simulink model "task4_lab10"  (R2021a)
settings: Solver=FixedStepDiscrete  StartTime=0.0  StopTime=10.0  RelTol=1e-3
settings Model: Creator=reemb  LastModifiedBy=reemb
settings OptimizationCC: DefaultParameterBehavior=Inlined  EnhancedBackFolding=on  PassReuseOutputArgsAs=Individual arguments  ZeroExternalMemoryAtStartup=off  ZeroInternalMemoryAtStartup=off  OptimizeBlockOrder=speed  DifferentSizesBufferReuse=on  OptimizationCustomize=off  EfficientTunableParamExpr=on
settings DebuggingCC: ParameterTunabilityLossMsg=error
settings SFSimCC: MATLABDynamicMemAlloc=off
settings RTWCC: SystemTargetFile=ert.tlc  GenCodeOnly=on  TemplateMakefile=ert_default_tmf
settings CodeAppCC: ForceParamTrailComments=on  IgnoreCustomStorageClasses=off  OperatorAnnotations=on  SimulinkDataObjDesc=on  SFDataObjDesc=on  InsertBlockDesc=on
settings ERTTargetCC: TargetLangStandard=C99 (ISO)  GenerateSampleERTMain=on  InlinedParameterPlacement=NonHierarchical  ERTCustomFileTemplate=example_file_process.tlc

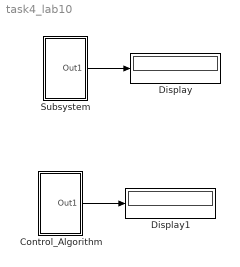
== system task4_lab10 ==
  Control_Algorithm : Subsystem  TreatAsAtomicUnit=on  RTWFcnName=algo_logic
      settings: RTWSystemCode=Nonreusable function  RTWFcnNameOpts=User specified  RTWFileNameOpts=Use function name
  Display : Display
  Display1 : Display
  Subsystem : Subsystem
  wires:
  Subsystem/1(Out1) -> Display/1
  Control_Algorithm/1(Out1) -> Display1/1

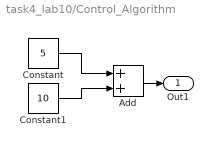
== system task4_lab10/Control_Algorithm ==
  Add : Sum
  Constant : Constant  Value=5
  Constant1 : Constant  Value=10
  Out1 : Outport
  wires:
  Constant/1 -> Add/1
  Add/1 -> Out1/1
  Constant1/1 -> Add/2

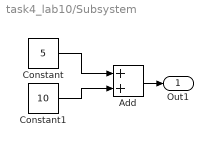
== system task4_lab10/Subsystem ==
  Add : Sum
  Constant : Constant  Value=5
  Constant1 : Constant  Value=10
  Out1 : Outport
  wires:
  Constant1/1 -> Add/2
  Add/1 -> Out1/1
  Constant/1 -> Add/1
